simulink model "sfcndemo_csfunc"  (Simulink 7.6)
settings: Solver=ode3  SolverMode=SingleTasking  StartTime=0.0  StopTime=10  FixedStep=.01  MaxStep=0.01  RelTol=1e-3  AbsTol=1e-6
Description:
  | Continuous-Time State-Space C-MEX S-function
settings Model: Creator=The MathWorks Inc.  ExtModeTrigMode=oneshot  ExtModeArmWhenConnect=off  ExtModeAutoUpdateStatusClock=off
settings DataIOCC: ExternalInput=[]  InitialState=[]  LimitDataPoints=off
settings OptimizationCC: BlockReduction=off  BooleanDataType=off  InitFltsAndDblsToZero=on
settings DebuggingCC: SaveWithParameterizedLinksMsg=none  SignalResolutionControl=TryResolveAllWithWarning  SolverPrmCheckMsg=none  InheritedTsInSrcMsg=none  MultiTaskDSMMsg=warning  MultiTaskCondExecSysMsg=none
settings HardwareCC: TargetUnknown=on
settings RTWCC: IncludeERTFirstTime=on
settings CodeAppCC: CustomSymbolStrFcn=$F$N$M
settings GRTTargetCC: TargetFcnLib=ansi_tfl_tmw.mat

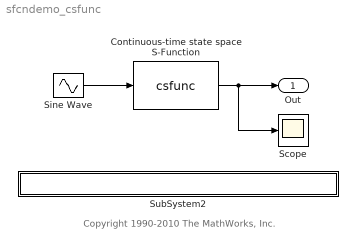
== system sfcndemo_csfunc ==
  note: Copyright 1990-2010 The MathWorks, Inc.
  Continuous-time state space S-Function : S-Function  FunctionName=csfunc  EnableBusSupport=off
      mask Type: S-function: csfunc
      mask Description: This is a S-function that does the continuous state space system.
      mask Display: disp('x'' = A*X + B*U\n Y = C*X + D*U ');
  Scope : Scope
      settings: TimeRange=10  YMin=-200  YMax=500
  Sine Wave : Sin  Amplitude=[1 2]  SampleTime=0
  SubSystem2 : Subsystem  mask{filename=csfunc.c}
      mask init:
      | x=sfundemo_maskdisp;
      settings: AttributesFormatString=\n  OpenFcn=sfundemo_openfcn
      mask Display: disp(x);
  Out : Outport  InitialOutput=0
  wires:
  Sine Wave/1 -> Continuous-time state space S-Function/1
  Continuous-time state space S-Function/1 -> Out/1, Scope/1

== system sfcndemo_csfunc/SubSystem2 ==
